simulink model "Simulation"  (R2022b)
settings: Solver=VariableStepAuto  StartTime=0.0  StopTime=1000  FixedStep=0.01  RelTol=1e-3
libraries: simulink x1
settings Model: Creator=Admin  LastModifiedBy=Admin

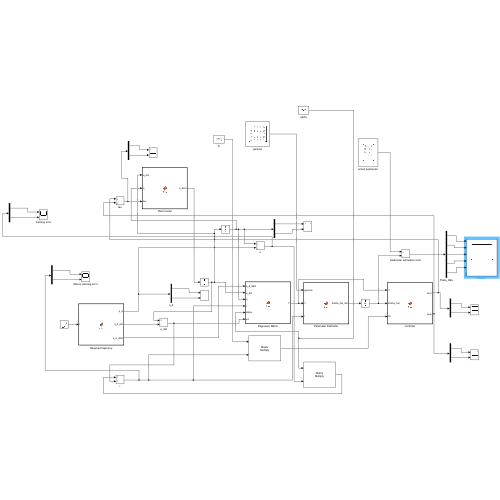
[thumbnail: Simulink's stored preview of the top-level diagram]
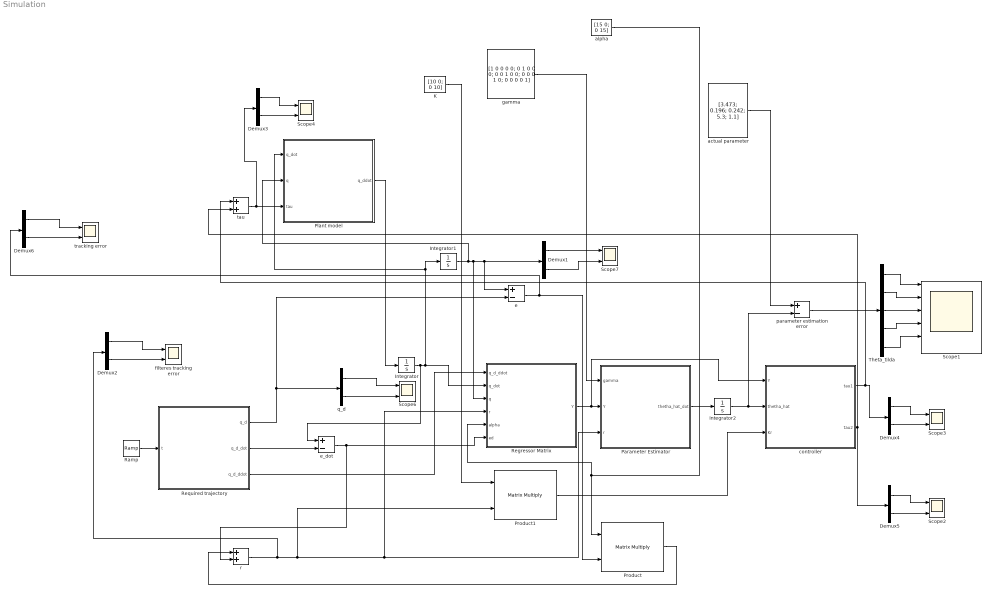
== system Simulation ==
  " tracking error" : Scope  NumInputPorts=2
  Demux{1..6} (6 alike) : Demux  Outputs=2
  Integrator : Integrator  InitialCondition=[0; 0]
  Integrator1 : Integrator  InitialCondition=[0; 0]
  Integrator2 : Integrator  InitialCondition=[0; 0; 0; 0; 0]
  K : Constant  Value=[10 0; 0 10]  VectorParams1D=off
  Parameter Estimator : MATLAB Function  TreatAsAtomicUnit=on
  Plant model : MATLAB Function  TreatAsAtomicUnit=on
  Product : Product  Multiplication=Matrix(*)
  Product1 : Product  Multiplication=Matrix(*)
  Ramp : simulink/Sources/Ramp  slope=1  start=0  InitialOutput=0
  Regressor Matrix : MATLAB Function  TreatAsAtomicUnit=on
  Required trajectory : MATLAB Function  TreatAsAtomicUnit=on
  Scope1 : Scope  NumInputPorts=6
  Scope{2..4,6..7} (5 alike) : Scope  NumInputPorts=2
  Theta_tilda : Demux  Outputs=5
  actual parameter : Constant  Value=[3.473; 0.196; 0.242; 5.3; 1.1]  VectorParams1D=off
  alpha : Constant  Value=[15 0; 0 15]  VectorParams1D=off
  controller : MATLAB Function  TreatAsAtomicUnit=on
  e : Sum  Inputs=+-
  e_dot : Sum  Inputs=+-
  filteres tracking error : Scope  NumInputPorts=2
  gamma : Constant  Value=[1 0 0 0 0; 0 1 0 0 0; 0 0 1 0 0; 0 0 0 1 0; 0 0 0 0 1]  VectorParams1D=off
  parameter estimation error : Sum  Inputs=+-
  q_d : Demux  Outputs=2
  r : Sum
  tau : Sum
  wires:
  Ramp/1 -> Required trajectory/1(t)
  Demux4/2 -> Scope3/2
  Integrator1/1 -> e/1, Demux1/1, Regressor Matrix/3(q), Plant model/2(q)
  Required trajectory/3(q_d_ddot) -> Regressor Matrix/1(q_d_ddot)
  Demux4/1 -> Scope3/1
  Required trajectory/1(q_d) -> q_d/1, e/2
  Required trajectory/2(q_d_dot) -> e_dot/2
  r/1 -> Demux2/1, Regressor Matrix/4(r), Parameter Estimator/3(r), Product1/2
  Demux5/2 -> Scope2/2
  Theta_tilda/4 -> Scope1/4
  Plant model/1(q_ddot) -> Integrator/1
  Demux1/2 -> Scope7/2
  q_d/1 -> Scope6/1
  Demux1/1 -> Scope7/1
  q_d/2 -> Scope6/2
  Demux5/1 -> Scope2/1
  e_dot/1 -> Regressor Matrix/6(ed), r/2
  Integrator2/1 -> controller/2(thetha_hat), parameter estimation error/2
  Integrator/1 -> Integrator1/1, Plant model/1(q_dot), Regressor Matrix/2(q_dot), e_dot/1
  K/1 -> Product1/1
  gamma/1 -> Parameter Estimator/1(gamma)
  Regressor Matrix/1(Y) -> controller/1(Y), Parameter Estimator/2(Y)
  Product1/1 -> controller/3(Kr)
  alpha/1 -> Product/1, Regressor Matrix/5(alpha)
  Parameter Estimator/1(thetha_hat_dot) -> Integrator2/1
  Product/1 -> r/1
  actual parameter/1 -> parameter estimation error/1
  parameter estimation error/1 -> Theta_tilda/1
  controller/1(tau1) -> tau/1, Demux4/1
  controller/2(tau2) -> tau/2, Demux5/1
  Theta_tilda/1 -> Scope1/1
  Theta_tilda/2 -> Scope1/2
  Theta_tilda/5 -> Scope1/5
  Theta_tilda/3 -> Scope1/3
  Demux2/1 -> filteres tracking error/1
  Demux2/2 -> filteres tracking error/2
  e/1 -> Demux6/1, Product/2
  Demux3/1 -> Scope4/1
  tau/1 -> Demux3/1, Plant model/3(tau)
  Demux3/2 -> Scope4/2
  Demux6/1 -> " tracking error"/1
  Demux6/2 -> " tracking error"/2

== matlab function Simulation/controller ==
  data: Y input size=2,5; thetha_hat input size=5,1; tau1 output size=2,1; Kr input; tau2 output
function [tau1, tau2] = fcn( Y, thetha_hat, Kr)
    tau1 = -Y*thetha_hat;
    tau2 = - Kr;

== matlab function Simulation/Plant model ==
  data: q_dot input size=2,1; q input size=2,1; q_ddot output size=2,1; tau input
function q_ddot = fcn(q_dot, q, tau)
p1 = 3.473;
p2 = 0.196;
p3 = 0.242;
fd1 = 5.3;
fd2 = 1.1;
c2 = cos(q(2));
s2 = sin(q(2));
M_q = [p1+2*p3*c2 p2+p3*c2; 
        p2+p3*c2 p2];
V_m =  [-p3*s2*q_dot(2) -p3*s2*(q_dot(1) + q_dot(2));
        p3*s2*q_dot(1) 0];
F_d = [fd1 0;
        0 fd2];
q_ddot = -(M_q)\(V_m*q_dot + F_d*q_dot) + tau;

== matlab function Simulation/Required trajectory ==
  data: q_d output; t input; q_d_dot output; q_d_ddot output
function [q_d, q_d_dot, q_d_ddot] = fcn(t)
q_d = [0.5*sin(t); 2*cos(t/4)];
q_d_dot = [0.5*cos(t); -0.5*sin(t/4)];
q_d_ddot = [-0.5*sin(t); -0.5*cos(t/4)/4];

== matlab function Simulation/Parameter Estimator ==
  data: gamma input; Y input; thetha_hat_dot output size=5,1; r input
function thetha_hat_dot = fcn( gamma, Y, r)
    thetha_hat_dot = gamma*(Y')*r;

== matlab function Simulation/Regressor Matrix ==
  data: q_d_ddot input; q_dot input size=2,1; q input; Y output; r input; alpha input; ed input
function Y = fcn( q_d_ddot, q_dot, q, r, alpha, ed)
    q2 = q(2);    
    s2 = sin(q2);
    c2 = cos(q2);
    qd1 = q_dot(1);
    qd2 = q_dot(2);
    qdd1 = q_d_ddot(1);
    qdd2 = q_d_ddot(2);
    r1 = r(1);
    r2 = r(2);
    a1 = alpha(1,1);
    a2 = alpha(2,2);
    ed1 = ed(1);
    ed2 = ed(2);
    
    A = [0          0               s2*qd1*qd2+s2*qd2*(qd1+qd2) 0       0;
         0          0               -s2*qd1*qd1                 0       0];

    B = [0          0               0                           -qd1    0;
         0          0               0                           0       -qd2];

    C = [-qdd1      -qdd2           -(2*c2*qdd1+c2*qdd2)        0       0;
         0          -(qdd1+qdd2)    -c2*qdd1                    0       0];

    D = [a1*ed1     a2*ed2          2*c2*a1*ed1+c2*a2*ed2       0       0;
         0          (a1*ed1+a2*ed2) (c2*a1*ed1)                 0       0];

    E = [0          0               -s2*r1*qd2-s2*r2*(qd1+qd2)  0       0;
         0          0               -s2*qd1*r1                  0       0];

    Y = A + B + C + D + E;
